simulink model "Transition"  (R2019a)
settings: Solver=VariableStepAuto  StartTime=0.0  StopTime=40  RelTol=1e-3
values from neighbouring files (symbols this model uses):
  agent = rlDDPGAgent(actor,critic,agentOptions)    [Agent.m]    (also in Bigger_Agent.m = agent.saved_agent; Multirotor_Agent.m = rlDDPGAgent(actor,critic,agentOpts); Transition_Agent.m = rlDDPGAgent(actor,critic,agentOpts))
  Ts = 0.4    [Agent.m]    (also in Bigger_Agent.m = 0.3; Multirotor_Agent.m = 0.3; Transition_Agent.m = 0.3)
libraries: simulink x14, simulink_extras x5, sharedutil x3, aerolibasang x2, shared6dof x1, aerolibadyn x1
(part 1 of 2)
settings Model: Creator=Michael  LastModifiedBy=admin
settings SolverCC: ZeroCrossAlgorithm=Adaptive
settings DebuggingCC: IgnoredZcDiagnostic=none

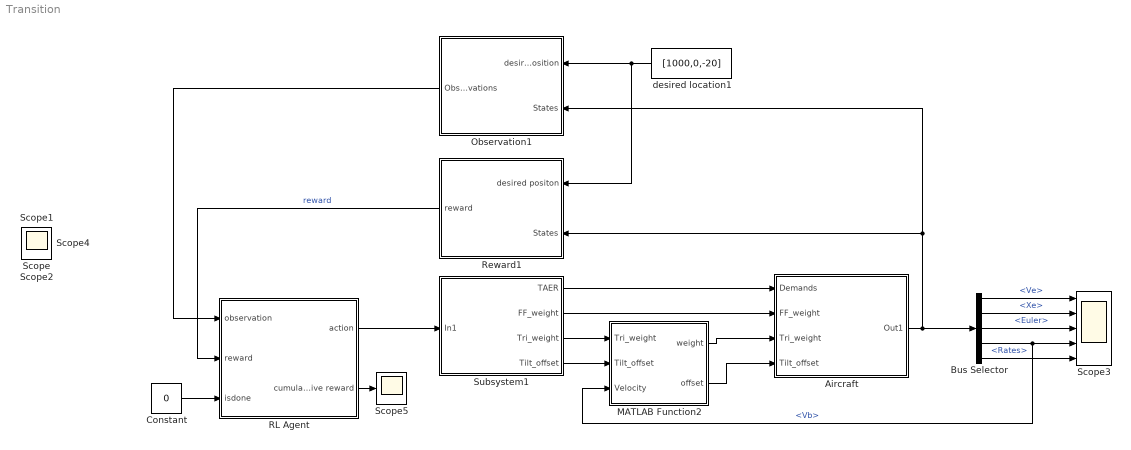
== system Transition ==
  "Aircraft " : Subsystem
  Bus Selector : BusSelector  OutputSignals=Ve,Xe,Euler,Vb,Rates
  Constant : Constant  Value=0
  MATLAB Function2 : MATLAB Function  TreatAsAtomicUnit=on
  Observation1 : Subsystem
  RL Agent : Subsystem  AncestorBlock=rllib/RL Agent  mask(RL Agent){Agent=agent, ProvideReward=on, ProvideIsDone=on, ProvideCumRwd=off, TreatAsDirectFeedthrough=on, CollectLoggedSignals=on, CollectModelStates=on}
      mask prompts: Agent "rl:block:RLAgentAgentPrompt"; ProvideReward "rl:block:RLAgentProvideRewardPrompt"; ProvideIsDone "rl:block:RLAgentProvideIsDonePrompt"; ProvideCumRwd "rl:block:RLAgentProvideCumRwdPrompt"; TreatAsDirectFeedthrough "rl:block:RLAgentDirectFeedthroughPrompt"; CollectLoggedSignals "rl:block:RLAgentCollectLoggedSignalsPrompt"; CollectModelStates "rl:block:RLAgentCollectModelStatesPrompt"
      mask help: rl:block:RLAgentDescription
      mask init:
      | agentmaskinit(gcb);
      mask Help: eval('rl.util.guihelp(''rlAgentBlock'')')
      mask DialogControl BDCollapsible Prompt: Block Diagram
      mask DialogControl AgentGroup Prompt: rl:block:RLAgentAgentGroupPrompt
      mask DialogControl Agent Prompt: Agent object
      mask DialogControl Agent Tooltip: rl:block:RLAgentAgentTooltip
      mask DialogControl PortGroup Prompt: rl:block:RLAgentPortsGroupPrompt
      mask DialogControl ProvideReward Prompt: Provide reward signal
      mask DialogControl ProvideReward Tooltip: rl:block:RLAgentProvideRewardTooltip
      mask DialogControl ProvideIsDone Prompt: Provide isdone signal
      mask DialogControl ProvideIsDone Tooltip: rl:block:RLAgentProvideIsDoneTooltip
      mask DialogControl ProvideCumRwd Prompt: Output cumulative reward signal
      mask DialogControl ProvideCumRwd Tooltip: rl:block:RLAgentProvideCumRwdTooltip
      mask DialogControl DirectFeedThroughGroup Prompt: rl:block:RLAgentDirectFeedthroughGroupPrompt
      mask DialogControl TreatAsDirectFeedthrough Prompt: Treat inputs as direct feedthrough
      mask DialogControl TreatAsDirectFeedthrough Tooltip: rl:block:RLAgentDirectFeedthroughTooltip
      mask DialogControl DataGroup Prompt: rl:block:RLAgentDataGroupPrompt
      mask DialogControl CollectLoggedSignals Prompt: Provide logged signals to agent
      mask DialogControl CollectLoggedSignals Tooltip: rl:block:RLAgentCollectLoggedSignalsTooltip
      mask DialogControl CollectModelStates Prompt: Provide model states to agent
      mask DialogControl CollectModelStates Tooltip: rl:block:RLAgentCollectModelStatesTooltip
  Reward1 : Subsystem
  Scope3 : Scope  NumInputPorts=5
  Scope{,1..2,4..5} (5 alike) : Scope
  Subsystem1 : Subsystem
  desired location1 : Constant  Value=[1000,0,-20]
  wires:
  Subsystem1/1(TAER) -> "Aircraft "/1(Demands)
  Bus Selector/1 -> Scope3/1  "<Ve>"
  Bus Selector/2 -> Scope3/2  "<Xe>"
  Bus Selector/3 -> Scope3/3  "<Euler>"
  Bus Selector/4 -> MATLAB Function2/3(Velocity), Scope3/4  "<Vb>"
  Bus Selector/5 -> Scope3/5  "<Rates>"
  RL Agent/1(action) -> Subsystem1/1(In1)
  Observation1/1("Observations ") -> RL Agent/1(observation)
  Reward1/1(reward) -> RL Agent/2(reward)  "reward"
  "Aircraft "/1(Out1) -> Bus Selector/1, Observation1/2(States), Reward1/2(States)
  Subsystem1/2(FF_weight) -> "Aircraft "/2(FF_weight)
  Subsystem1/3(Tri_weight) -> MATLAB Function2/1(Tri_weight)
  Subsystem1/4(Tilt_offset) -> MATLAB Function2/2(Tilt_offset)
  MATLAB Function2/1(weight) -> "Aircraft "/3(Tri_weight)
  MATLAB Function2/2(offset) -> "Aircraft "/4(Tilt_offset)
  Constant/1 -> RL Agent/3(isdone)
  RL Agent/2(cumulative reward) -> Scope5/1
  desired location1/1 -> Reward1/1(desired positon), Observation1/1(desired position)

== system Transition/Aircraft  ==
  Demands : Inport
  FF_weight : Inport  Port=2
  Tri_weight : Inport  Port=3
  Tilt_offset : Inport  Port=4
  FFController1 : Subsystem
  FF_Attitude Controller1 : Subsystem
  Flight Dynamics : Subsystem  mask{mass=7}
  Subsystem1 : Subsystem
  Tri_Attitude Controller : Subsystem
  Tri_Rates_Controller : Subsystem
  Out1 : Outport
  wires:
  Flight Dynamics/1(States) -> Tri_Attitude Controller/2("States "), FF_Attitude Controller1/2("States "), Tri_Rates_Controller/2("States "), FFController1/2("States "), Out1/1
  Tri_Rates_Controller/1(Control) -> Subsystem1/5(Tri Control)
  Tri_Attitude Controller/1(Rate Demand) -> Tri_Rates_Controller/1(Demand)
  Subsystem1/1(Out1) -> Flight Dynamics/1(Control)
  FFController1/1(Control) -> Subsystem1/1(FF Control)
  FF_weight/1 -> Subsystem1/2(FF Weight)
  Tri_weight/1 -> Subsystem1/3("Tri Weight ")
  FF_Attitude Controller1/1(Rate Demand) -> FFController1/1(Demand)
  Demands/1 -> Tri_Attitude Controller/1("Demand "), FF_Attitude Controller1/1("Demand ")
  Tilt_offset/1 -> Subsystem1/4(Tilt_offset)

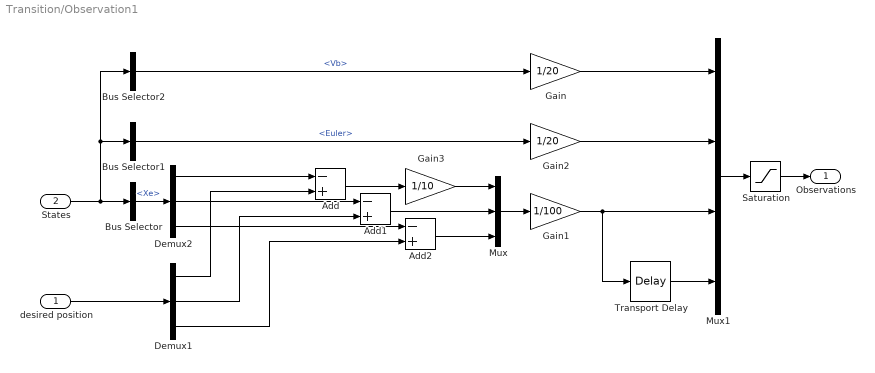
== system Transition/Observation1 ==
  desired position : Inport
  States : Inport  Port=2
  Add : Sum  Inputs=-+
  Add1 : Sum  Inputs=-+
  Add2 : Sum  Inputs=-+
  Bus Selector : BusSelector  OutputSignals=Xe
  Bus Selector1 : BusSelector  OutputSignals=Euler
  Bus Selector2 : BusSelector  OutputSignals=Vb
  Demux1 : Demux  Outputs=3
  Demux2 : Demux  Outputs=3
  Gain : Gain  Gain=1/20
  Gain1 : Gain  Gain=1/100
  Gain2 : Gain  Gain=1/20
  Gain3 : Gain  Gain=1/10
  Mux : Mux  Inputs=3
  Mux1 : Mux
  Saturation : Saturate  UpperLimit=1  LowerLimit=-1
  Transport Delay : TransportDelay  DelayTime=Ts
  "Observations " : Outport
  wires:
  desired position/1 -> Demux1/1
  Mux1/1 -> Saturation/1
  Add/1 -> Gain3/1
  Demux1/3 -> Add2/2
  Add2/1 -> Mux/3
  Add1/1 -> Mux/2
  Demux2/3 -> Add2/1
  Bus Selector/1 -> Demux2/1  "<Xe>"
  Demux1/2 -> Add1/2
  Demux2/1 -> Add/1
  Demux2/2 -> Add1/1
  Demux1/1 -> Add/2
  Bus Selector1/1 -> Gain2/1  "<Euler>"
  States/1 -> Bus Selector2/1, Bus Selector1/1, Bus Selector/1
  Bus Selector2/1 -> Gain/1  "<Vb>"
  Mux/1 -> Gain1/1
  Gain/1 -> Mux1/1
  Gain2/1 -> Mux1/2
  Gain1/1 -> Transport Delay/1, Mux1/3
  Transport Delay/1 -> Mux1/4
  Saturation/1 -> "Observations "/1
  Gain3/1 -> Mux/1

== system Transition/RL Agent ==
  observation : Inport
  reward : Inport  Port=2
  isdone : Inport  Port=3
  AgentWrapper : MATLABSystem  System=AgentWrapper  ModelName=Transition  AgentObjectName=Agent  BlockPath=Transition/RL Agent/AgentWrapper  TreatAsDirectFeedthrough=true  IsRewardProvided=true  IsIsDoneProvided=true  CollectLoggedSignals=true  CollectModelStates=true
      mask Type: AgentWrapper
      mask Display:
      | disp('AgentWrapper');
      | port_label('input',1,'observation');
      | port_label('input',2,'reward');
      | port_label('input',3,'isdone');
      | port_label('output',1,'action');
  accumulate_reward : Subsystem
  cumulative_reward : Terminator
  action : Outport
  cumulative reward : Outport  Port=2
  wires:
  AgentWrapper/1 -> action/1
  accumulate_reward/1(cumulative_reward) -> cumulative_reward/1, cumulative reward/1
  observation/1 -> AgentWrapper/1
  reward/1 -> accumulate_reward/1(reward), AgentWrapper/2
  isdone/1 -> AgentWrapper/3

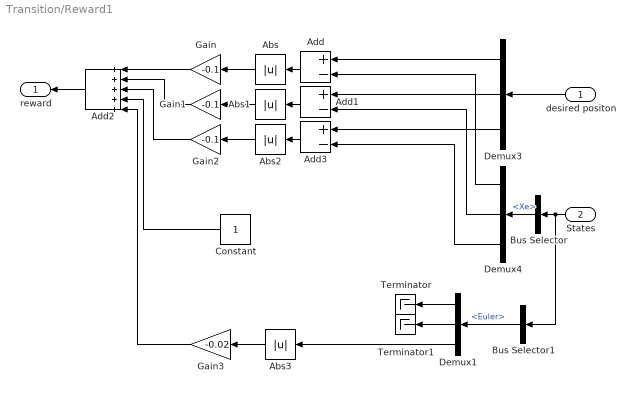
== system Transition/Reward1 ==
  desired positon : Inport
  States : Inport  Port=2
  Abs{,1..3} (4 alike) : Abs
  Add : Sum  Inputs=+-
  Add1 : Sum  Inputs=+-
  Add2 : Sum  Inputs=+++++
  Add3 : Sum  Inputs=+-
  Bus Selector : BusSelector  OutputSignals=Xe
  Bus Selector1 : BusSelector  OutputSignals=Euler
  Constant : Constant
  Demux1 : Demux  Outputs=3
  Demux3 : Demux  Outputs=3
  Demux4 : Demux  Outputs=3
  Gain : Gain  Gain=-0.1
  Gain1 : Gain  Gain=-0.1
  Gain2 : Gain  Gain=-0.1
  Gain3 : Gain  Gain=-0.02
  Terminator : Terminator
  Terminator1 : Terminator
  reward : Outport
  wires:
  Demux3/1 -> Add/1
  desired positon/1 -> Demux3/1
  Bus Selector/1 -> Demux4/1  "<Xe>"
  Add/1 -> Abs/1
  Demux4/1 -> Add/2
  Abs/1 -> Gain/1
  Demux3/2 -> Add1/1
  Demux4/2 -> Add1/2
  Abs1/1 -> Gain1/1
  Add1/1 -> Abs1/1
  Gain1/1 -> Add2/2
  Gain/1 -> Add2/1
  Add2/1 -> reward/1
  Gain2/1 -> Add2/3
  Add3/1 -> Abs2/1
  Abs2/1 -> Gain2/1
  Demux3/3 -> Add3/1
  Demux4/3 -> Add3/2
  Constant/1 -> Add2/4
  Bus Selector1/1 -> Demux1/1  "<Euler>"
  States/1 -> Bus Selector1/1, Bus Selector/1
  Demux1/1 -> Terminator/1
  Demux1/2 -> Terminator1/1
  Demux1/3 -> Abs3/1
  Abs3/1 -> Gain3/1
  Gain3/1 -> Add2/5

== system Transition/Subsystem1 ==
  In1 : Inport
  -1/1 to 0/1_1 : Subsystem
  -1/1 to 0/1_2 : Subsystem
  -1/1 to 0/1_3 : Subsystem
  Bus Creator : BusCreator  Inputs=4
  Constant : Constant  Value=0
  Demux1 : Demux  Outputs=6
  Gain4 : Gain  Gain=90
  TAER : Outport
  FF_weight : Outport  Port=2
  Tri_weight : Outport  Port=3
  Tilt_offset : Outport  Port=4
  wires:
  Demux1/2 -> Bus Creator/3  "Rd"
  Demux1/1 -> Bus Creator/2  "Xv"
  Demux1/3 -> Bus Creator/4  "Pd"
  -1/1 to 0/1_1/1(o) -> Gain4/1
  -1/1 to 0/1_3/1(o) -> FF_weight/1
  Gain4/1 -> Tilt_offset/1
  In1/1 -> Demux1/1
  Demux1/4 -> -1/1 to 0/1_1/1(<i>)
  Demux1/5 -> -1/1 to 0/1_2/1(<i>)
  Demux1/6 -> -1/1 to 0/1_3/1(<i>)
  -1/1 to 0/1_2/1(o) -> Tri_weight/1
  Constant/1 -> Bus Creator/1  "Yd"
  Bus Creator/1 -> TAER/1

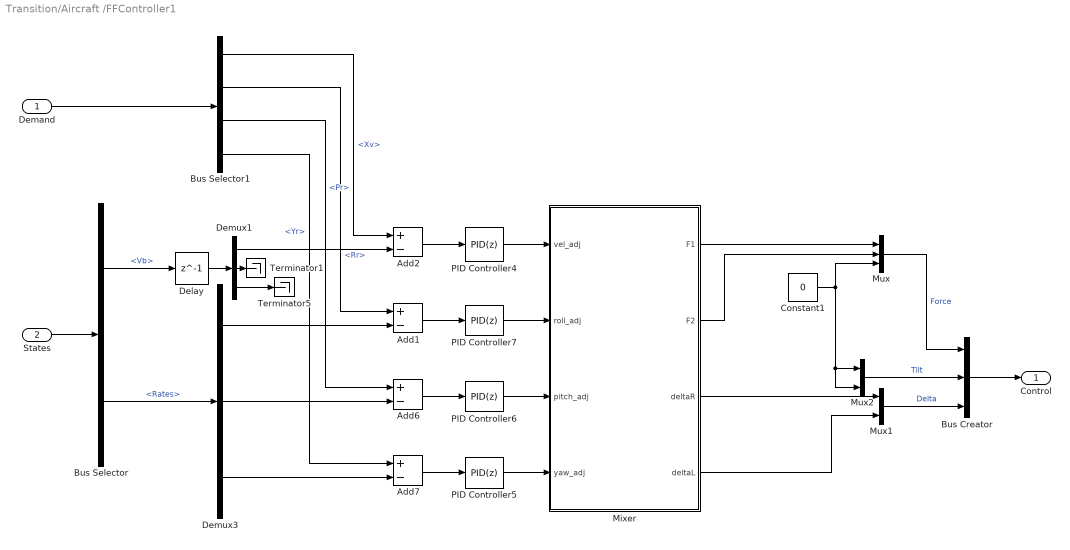
== system Transition/Aircraft /FFController1 ==
  Demand : Inport
  "States " : Inport  Port=2
  Add{1..2,6..7} (4 alike) : Sum  Inputs=+-
  Bus Creator : BusCreator  Inputs=3
  Bus Selector : BusSelector  OutputSignals=Vb,Rates
  Bus Selector1 : BusSelector  OutputSignals=Xv,Rr,Pr,Yr
  Constant1 : Constant  Value=0
  Delay : Delay  DelayLength=1  InitialCondition=0
  Demux1 : Demux  Outputs=3
  Demux3 : Demux  Outputs=3
  Mixer : Subsystem
  Mux : Mux  Inputs=3
  Mux1 : Mux  Inputs=2
  Mux2 : Mux  Inputs=2
  PID Controller4 : simulink/Continuous/PID Controller  Controller=PID  Form=Parallel  TimeDomain=Discrete-time  SampleTime=0.001  IntegratorMethod=Forward Euler  FilterMethod=Forward Euler  ControllerParametersSource=internal  P=30  I=0  D=1  UseFilter=on  N=21.8158810168648  TunerSelectOption=Transfer Function Based (PID Tuner App)  InitialConditionSource=internal  InitialConditionForIntegrator=0  InitialConditionForFilter=0  DifferentiatorICPrevScaledInput=0  ExternalReset=none  TrackingMode=off  Kt=1  LimitOutput=off  UpperSaturationLimit=inf  LowerSaturationLimit=-inf  LinearizeAsGain=on  AntiWindupMode=none  Kb=1  POutMin=[]  POutMax=[]  IOutMin=[]  IOutMax=[]  DOutMin=[]  DOutMax=[]  NOutMin=[]  NOutMax=[]  SumOutMin=[]  SumOutMax=[]  SaturationOutMin=[]  SaturationOutMax=[]  PParamMin=[]  PParamMax=[]  IParamMin=[]  IParamMax=[]  DParamMin=[]  DParamMax=[]  NParamMin=[]  NParamMax=[]  KbParamMin=[]  KbParamMax=[]  KtParamMin=[]  KtParamMax=[]  KbOutMin=[]  KbOutMax=[]  KtOutMin=[]  KtOutMax=[]  IntegratorOutMin=[]  IntegratorOutMax=[]  FilterOutMin=[]  FilterOutMax=[]  SumI1OutMin=[]  SumI1OutMax=[]  SumI2OutMin=[]  SumI2OutMax=[]  SumI3OutMin=[]  SumI3OutMax=[]  SumI4OutMin=[]  SumI4OutMax=[]  SumDOutMin=[]  SumDOutMax=[]  DifferentiatorOutMin=[]  DifferentiatorOutMax=[]  FilterDiffOutCoefMin=[]  FilterDiffOutCoefMax=[]  ReciprocalOutMin=[]  ReciprocalOutMax=[]  SumDenOutMin=[]  SumDenOutMax=[]  SumNumOutMin=[]  SumNumOutMax=[]  DivideOutMin=[]  DivideOutMax=[]  IntegratorContinuousStateAttributes=''  IntegratorStateMustResolveToSignalObject=off  IntegratorRTWStateStorageClass=Auto  FilterContinuousStateAttributes=''  FilterStateMustResolveToSignalObject=off  FilterRTWStateStorageClass=Auto  ParallelPVariant=InternalParameters  IdealPVariant=Disabled  IVariant=InternalParameters  DVariant=InternalParameters  IntegratorVariant=Discrete  SatVariant=Disabled  AWVariant=Passthrough  PCopyVariant=Disabled  TRVariant=Disabled  FdbkBlocksVariant=Forward  IdealPFdbkVariant=Disabled  SatFdbkVariant=Disabled  DerivativeFilterVariant=ForwardEulerFilter  NVariant=InternalParameters  NCopyVariant=Disabled  FilterICVariant=InternalICsFilter  IntegratorICVariant=InternalICs  ExternalResetVariant=Disabled  TRSumVariant=Passthrough  SumFdbkVariant=Disabled  SumVariant=Sum_PID
  PID Controller5 : simulink/Continuous/PID Controller  Controller=PID  Form=Parallel  TimeDomain=Discrete-time  SampleTime=0.001  IntegratorMethod=Forward Euler  FilterMethod=Forward Euler  ControllerParametersSource=internal  P=30  I=0.01  D=2  UseFilter=on  N=200  TunerSelectOption=Transfer Function Based (PID Tuner App)  InitialConditionSource=internal  InitialConditionForIntegrator=0  InitialConditionForFilter=0  DifferentiatorICPrevScaledInput=0  ExternalReset=none  TrackingMode=off  Kt=1  LimitOutput=off  UpperSaturationLimit=inf  LowerSaturationLimit=-inf  LinearizeAsGain=on  AntiWindupMode=none  Kb=1  POutMin=[]  POutMax=[]  IOutMin=[]  IOutMax=[]  DOutMin=[]  DOutMax=[]  NOutMin=[]  NOutMax=[]  SumOutMin=[]  SumOutMax=[]  SaturationOutMin=[]  SaturationOutMax=[]  PParamMin=[]  PParamMax=[]  IParamMin=[]  IParamMax=[]  DParamMin=[]  DParamMax=[]  NParamMin=[]  NParamMax=[]  KbParamMin=[]  KbParamMax=[]  KtParamMin=[]  KtParamMax=[]  KbOutMin=[]  KbOutMax=[]  KtOutMin=[]  KtOutMax=[]  IntegratorOutMin=[]  IntegratorOutMax=[]  FilterOutMin=[]  FilterOutMax=[]  SumI1OutMin=[]  SumI1OutMax=[]  SumI2OutMin=[]  SumI2OutMax=[]  SumI3OutMin=[]  SumI3OutMax=[]  SumI4OutMin=[]  SumI4OutMax=[]  SumDOutMin=[]  SumDOutMax=[]  DifferentiatorOutMin=[]  DifferentiatorOutMax=[]  FilterDiffOutCoefMin=[]  FilterDiffOutCoefMax=[]  ReciprocalOutMin=[]  ReciprocalOutMax=[]  SumDenOutMin=[]  SumDenOutMax=[]  SumNumOutMin=[]  SumNumOutMax=[]  DivideOutMin=[]  DivideOutMax=[]  IntegratorContinuousStateAttributes=''  IntegratorStateMustResolveToSignalObject=off  IntegratorRTWStateStorageClass=Auto  FilterContinuousStateAttributes=''  FilterStateMustResolveToSignalObject=off  FilterRTWStateStorageClass=Auto  ParallelPVariant=InternalParameters  IdealPVariant=Disabled  IVariant=InternalParameters  DVariant=InternalParameters  IntegratorVariant=Discrete  SatVariant=Disabled  AWVariant=Passthrough  PCopyVariant=Disabled  TRVariant=Disabled  FdbkBlocksVariant=Forward  IdealPFdbkVariant=Disabled  SatFdbkVariant=Disabled  DerivativeFilterVariant=ForwardEulerFilter  NVariant=InternalParameters  NCopyVariant=Disabled  FilterICVariant=InternalICsFilter  IntegratorICVariant=InternalICs  ExternalResetVariant=Disabled  TRSumVariant=Passthrough  SumFdbkVariant=Disabled  SumVariant=Sum_PID
  PID Controller6 : simulink/Continuous/PID Controller  Controller=PID  Form=Parallel  TimeDomain=Discrete-time  SampleTime=0.001  IntegratorMethod=Forward Euler  FilterMethod=Forward Euler  ControllerParametersSource=internal  P=40  I=0.01  D=2  UseFilter=on  N=200  TunerSelectOption=Transfer Function Based (PID Tuner App)  InitialConditionSource=internal  InitialConditionForIntegrator=0  InitialConditionForFilter=0  DifferentiatorICPrevScaledInput=0  ExternalReset=none  TrackingMode=off  Kt=1  LimitOutput=off  UpperSaturationLimit=inf  LowerSaturationLimit=-inf  LinearizeAsGain=on  AntiWindupMode=none  Kb=1  POutMin=[]  POutMax=[]  IOutMin=[]  IOutMax=[]  DOutMin=[]  DOutMax=[]  NOutMin=[]  NOutMax=[]  SumOutMin=[]  SumOutMax=[]  SaturationOutMin=[]  SaturationOutMax=[]  PParamMin=[]  PParamMax=[]  IParamMin=[]  IParamMax=[]  DParamMin=[]  DParamMax=[]  NParamMin=[]  NParamMax=[]  KbParamMin=[]  KbParamMax=[]  KtParamMin=[]  KtParamMax=[]  KbOutMin=[]  KbOutMax=[]  KtOutMin=[]  KtOutMax=[]  IntegratorOutMin=[]  IntegratorOutMax=[]  FilterOutMin=[]  FilterOutMax=[]  SumI1OutMin=[]  SumI1OutMax=[]  SumI2OutMin=[]  SumI2OutMax=[]  SumI3OutMin=[]  SumI3OutMax=[]  SumI4OutMin=[]  SumI4OutMax=[]  SumDOutMin=[]  SumDOutMax=[]  DifferentiatorOutMin=[]  DifferentiatorOutMax=[]  FilterDiffOutCoefMin=[]  FilterDiffOutCoefMax=[]  ReciprocalOutMin=[]  ReciprocalOutMax=[]  SumDenOutMin=[]  SumDenOutMax=[]  SumNumOutMin=[]  SumNumOutMax=[]  DivideOutMin=[]  DivideOutMax=[]  IntegratorContinuousStateAttributes=''  IntegratorStateMustResolveToSignalObject=off  IntegratorRTWStateStorageClass=Auto  FilterContinuousStateAttributes=''  FilterStateMustResolveToSignalObject=off  FilterRTWStateStorageClass=Auto  ParallelPVariant=InternalParameters  IdealPVariant=Disabled  IVariant=InternalParameters  DVariant=InternalParameters  IntegratorVariant=Discrete  SatVariant=Disabled  AWVariant=Passthrough  PCopyVariant=Disabled  TRVariant=Disabled  FdbkBlocksVariant=Forward  IdealPFdbkVariant=Disabled  SatFdbkVariant=Disabled  DerivativeFilterVariant=ForwardEulerFilter  NVariant=InternalParameters  NCopyVariant=Disabled  FilterICVariant=InternalICsFilter  IntegratorICVariant=InternalICs  ExternalResetVariant=Disabled  TRSumVariant=Passthrough  SumFdbkVariant=Disabled  SumVariant=Sum_PID
  PID Controller7 : simulink/Continuous/PID Controller  Controller=PID  Form=Parallel  TimeDomain=Discrete-time  SampleTime=0.001  IntegratorMethod=Forward Euler  FilterMethod=Forward Euler  ControllerParametersSource=internal  P=20  I=0.01  D=2  UseFilter=on  N=200  TunerSelectOption=Transfer Function Based (PID Tuner App)  InitialConditionSource=internal  InitialConditionForIntegrator=0  InitialConditionForFilter=0  DifferentiatorICPrevScaledInput=0  ExternalReset=none  TrackingMode=off  Kt=1  LimitOutput=off  UpperSaturationLimit=inf  LowerSaturationLimit=-inf  LinearizeAsGain=on  AntiWindupMode=none  Kb=1  POutMin=[]  POutMax=[]  IOutMin=[]  IOutMax=[]  DOutMin=[]  DOutMax=[]  NOutMin=[]  NOutMax=[]  SumOutMin=[]  SumOutMax=[]  SaturationOutMin=[]  SaturationOutMax=[]  PParamMin=[]  PParamMax=[]  IParamMin=[]  IParamMax=[]  DParamMin=[]  DParamMax=[]  NParamMin=[]  NParamMax=[]  KbParamMin=[]  KbParamMax=[]  KtParamMin=[]  KtParamMax=[]  KbOutMin=[]  KbOutMax=[]  KtOutMin=[]  KtOutMax=[]  IntegratorOutMin=[]  IntegratorOutMax=[]  FilterOutMin=[]  FilterOutMax=[]  SumI1OutMin=[]  SumI1OutMax=[]  SumI2OutMin=[]  SumI2OutMax=[]  SumI3OutMin=[]  SumI3OutMax=[]  SumI4OutMin=[]  SumI4OutMax=[]  SumDOutMin=[]  SumDOutMax=[]  DifferentiatorOutMin=[]  DifferentiatorOutMax=[]  FilterDiffOutCoefMin=[]  FilterDiffOutCoefMax=[]  ReciprocalOutMin=[]  ReciprocalOutMax=[]  SumDenOutMin=[]  SumDenOutMax=[]  SumNumOutMin=[]  SumNumOutMax=[]  DivideOutMin=[]  DivideOutMax=[]  IntegratorContinuousStateAttributes=''  IntegratorStateMustResolveToSignalObject=off  IntegratorRTWStateStorageClass=Auto  FilterContinuousStateAttributes=''  FilterStateMustResolveToSignalObject=off  FilterRTWStateStorageClass=Auto  ParallelPVariant=InternalParameters  IdealPVariant=Disabled  IVariant=InternalParameters  DVariant=InternalParameters  IntegratorVariant=Discrete  SatVariant=Disabled  AWVariant=Passthrough  PCopyVariant=Disabled  TRVariant=Disabled  FdbkBlocksVariant=Forward  IdealPFdbkVariant=Disabled  SatFdbkVariant=Disabled  DerivativeFilterVariant=ForwardEulerFilter  NVariant=InternalParameters  NCopyVariant=Disabled  FilterICVariant=InternalICsFilter  IntegratorICVariant=InternalICs  ExternalResetVariant=Disabled  TRSumVariant=Passthrough  SumFdbkVariant=Disabled  SumVariant=Sum_PID
  Terminator1 : Terminator
  Terminator5 : Terminator
  Control : Outport
  wires:
  Mixer/1(F1) -> Mux/1
  Mixer/2(F2) -> Mux/2
  Mixer/3(deltaR) -> Mux1/1
  Mixer/4(deltaL) -> Mux1/2
  Mux1/1 -> Bus Creator/3  "Delta"
  Mux/1 -> Bus Creator/1  "Force"
  Constant1/1 -> Mux2/2, Mux2/1, Mux/3
  Mux2/1 -> Bus Creator/2  "Tilt"
  Bus Creator/1 -> Control/1
  PID Controller7/1 -> Mixer/2(roll_adj)
  Add1/1 -> PID Controller7/1
  Bus Selector1/3 -> Add6/1  "<Pr>"
  Add6/1 -> PID Controller6/1
  PID Controller6/1 -> Mixer/3(pitch_adj)
  Add7/1 -> PID Controller5/1
  Bus Selector1/4 -> Add7/1  "<Yr>"
  Demux3/2 -> Add6/2
  Demux1/1 -> Add2/2
  Demux1/2 -> Terminator1/1
  Bus Selector/2 -> Demux3/1  "<Rates>"
  Bus Selector1/2 -> Add1/1  "<Rr>"
  Bus Selector/1 -> Delay/1  "<Vb>"
  Add2/1 -> PID Controller4/1
  Demux3/3 -> Add7/2
  PID Controller5/1 -> Mixer/4(yaw_adj)
  PID Controller4/1 -> Mixer/1(vel_adj)
  Demux3/1 -> Add1/2
  Demand/1 -> Bus Selector1/1
  Bus Selector1/1 -> Add2/1  "<Xv>"
  "States "/1 -> Bus Selector/1
  Demux1/3 -> Terminator5/1
  Delay/1 -> Demux1/1

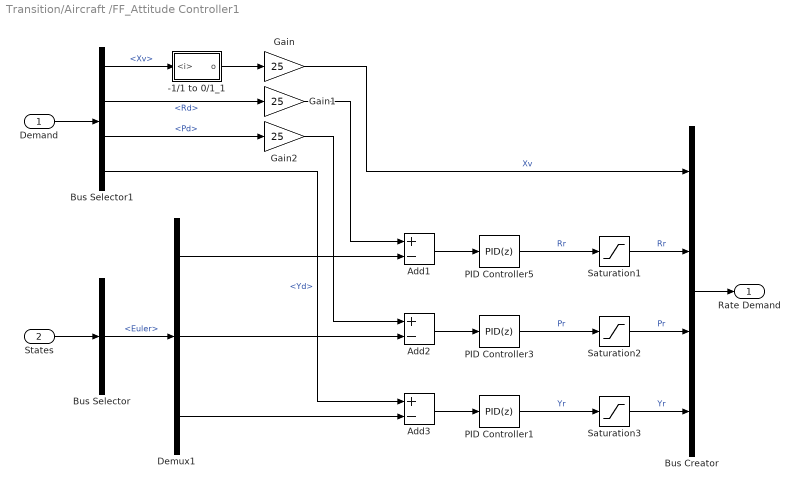
== system Transition/Aircraft /FF_Attitude Controller1 ==
  "Demand " : Inport
  "States " : Inport  Port=2
  -1/1 to 0/1_1 : Subsystem
  Add1 : Sum  Inputs=+-
  Add2 : Sum  Inputs=+-
  Add3 : Sum  Inputs=+-
  Bus Creator : BusCreator  Inputs=4
  Bus Selector : BusSelector  OutputSignals=Euler
  Bus Selector1 : BusSelector  OutputSignals=Xv,Rd,Pd,Yd
  Demux1 : Demux  Outputs=3
  Gain : Gain  Gain=25
  Gain1 : Gain  Gain=25
  Gain2 : Gain  Gain=25
  PID Controller1 : simulink/Continuous/PID Controller  Controller=PID  Form=Parallel  TimeDomain=Discrete-time  SampleTime=0.001  IntegratorMethod=Forward Euler  FilterMethod=Forward Euler  ControllerParametersSource=internal  P=3  I=0  D=0  UseFilter=on  N=200  TunerSelectOption=Transfer Function Based (PID Tuner App)  InitialConditionSource=internal  InitialConditionForIntegrator=0  InitialConditionForFilter=0  DifferentiatorICPrevScaledInput=0  ExternalReset=none  TrackingMode=off  Kt=1  LimitOutput=off  UpperSaturationLimit=inf  LowerSaturationLimit=-inf  LinearizeAsGain=on  AntiWindupMode=none  Kb=1  POutMin=[]  POutMax=[]  IOutMin=[]  IOutMax=[]  DOutMin=[]  DOutMax=[]  NOutMin=[]  NOutMax=[]  SumOutMin=[]  SumOutMax=[]  SaturationOutMin=[]  SaturationOutMax=[]  PParamMin=[]  PParamMax=[]  IParamMin=[]  IParamMax=[]  DParamMin=[]  DParamMax=[]  NParamMin=[]  NParamMax=[]  KbParamMin=[]  KbParamMax=[]  KtParamMin=[]  KtParamMax=[]  KbOutMin=[]  KbOutMax=[]  KtOutMin=[]  KtOutMax=[]  IntegratorOutMin=[]  IntegratorOutMax=[]  FilterOutMin=[]  FilterOutMax=[]  SumI1OutMin=[]  SumI1OutMax=[]  SumI2OutMin=[]  SumI2OutMax=[]  SumI3OutMin=[]  SumI3OutMax=[]  SumI4OutMin=[]  SumI4OutMax=[]  SumDOutMin=[]  SumDOutMax=[]  DifferentiatorOutMin=[]  DifferentiatorOutMax=[]  FilterDiffOutCoefMin=[]  FilterDiffOutCoefMax=[]  ReciprocalOutMin=[]  ReciprocalOutMax=[]  SumDenOutMin=[]  SumDenOutMax=[]  SumNumOutMin=[]  SumNumOutMax=[]  DivideOutMin=[]  DivideOutMax=[]  IntegratorContinuousStateAttributes=''  IntegratorStateMustResolveToSignalObject=off  IntegratorRTWStateStorageClass=Auto  FilterContinuousStateAttributes=''  FilterStateMustResolveToSignalObject=off  FilterRTWStateStorageClass=Auto  ParallelPVariant=InternalParameters  IdealPVariant=Disabled  IVariant=InternalParameters  DVariant=InternalParameters  IntegratorVariant=Discrete  SatVariant=Disabled  AWVariant=Passthrough  PCopyVariant=Disabled  TRVariant=Disabled  FdbkBlocksVariant=Forward  IdealPFdbkVariant=Disabled  SatFdbkVariant=Disabled  DerivativeFilterVariant=ForwardEulerFilter  NVariant=InternalParameters  NCopyVariant=Disabled  FilterICVariant=InternalICsFilter  IntegratorICVariant=InternalICs  ExternalResetVariant=Disabled  TRSumVariant=Passthrough  SumFdbkVariant=Disabled  SumVariant=Sum_PID
  PID Controller3 : simulink/Continuous/PID Controller  Controller=PID  Form=Parallel  TimeDomain=Discrete-time  SampleTime=0.001  IntegratorMethod=Forward Euler  FilterMethod=Forward Euler  ControllerParametersSource=internal  P=40  I=0.1  D=0.5  UseFilter=on  N=200  TunerSelectOption=Transfer Function Based (PID Tuner App)  InitialConditionSource=internal  InitialConditionForIntegrator=0  InitialConditionForFilter=0  DifferentiatorICPrevScaledInput=0  ExternalReset=none  TrackingMode=off  Kt=1  LimitOutput=off  UpperSaturationLimit=inf  LowerSaturationLimit=-inf  LinearizeAsGain=on  AntiWindupMode=none  Kb=1  POutMin=[]  POutMax=[]  IOutMin=[]  IOutMax=[]  DOutMin=[]  DOutMax=[]  NOutMin=[]  NOutMax=[]  SumOutMin=[]  SumOutMax=[]  SaturationOutMin=[]  SaturationOutMax=[]  PParamMin=[]  PParamMax=[]  IParamMin=[]  IParamMax=[]  DParamMin=[]  DParamMax=[]  NParamMin=[]  NParamMax=[]  KbParamMin=[]  KbParamMax=[]  KtParamMin=[]  KtParamMax=[]  KbOutMin=[]  KbOutMax=[]  KtOutMin=[]  KtOutMax=[]  IntegratorOutMin=[]  IntegratorOutMax=[]  FilterOutMin=[]  FilterOutMax=[]  SumI1OutMin=[]  SumI1OutMax=[]  SumI2OutMin=[]  SumI2OutMax=[]  SumI3OutMin=[]  SumI3OutMax=[]  SumI4OutMin=[]  SumI4OutMax=[]  SumDOutMin=[]  SumDOutMax=[]  DifferentiatorOutMin=[]  DifferentiatorOutMax=[]  FilterDiffOutCoefMin=[]  FilterDiffOutCoefMax=[]  ReciprocalOutMin=[]  ReciprocalOutMax=[]  SumDenOutMin=[]  SumDenOutMax=[]  SumNumOutMin=[]  SumNumOutMax=[]  DivideOutMin=[]  DivideOutMax=[]  IntegratorContinuousStateAttributes=''  IntegratorStateMustResolveToSignalObject=off  IntegratorRTWStateStorageClass=Auto  FilterContinuousStateAttributes=''  FilterStateMustResolveToSignalObject=off  FilterRTWStateStorageClass=Auto  ParallelPVariant=InternalParameters  IdealPVariant=Disabled  IVariant=InternalParameters  DVariant=InternalParameters  IntegratorVariant=Discrete  SatVariant=Disabled  AWVariant=Passthrough  PCopyVariant=Disabled  TRVariant=Disabled  FdbkBlocksVariant=Forward  IdealPFdbkVariant=Disabled  SatFdbkVariant=Disabled  DerivativeFilterVariant=ForwardEulerFilter  NVariant=InternalParameters  NCopyVariant=Disabled  FilterICVariant=InternalICsFilter  IntegratorICVariant=InternalICs  ExternalResetVariant=Disabled  TRSumVariant=Passthrough  SumFdbkVariant=Disabled  SumVariant=Sum_PID
  PID Controller5 : simulink/Continuous/PID Controller  Controller=PID  Form=Parallel  TimeDomain=Discrete-time  SampleTime=0.001  IntegratorMethod=Forward Euler  FilterMethod=Forward Euler  ControllerParametersSource=internal  P=20  I=0.1  D=0.5  UseFilter=on  N=200  TunerSelectOption=Transfer Function Based (PID Tuner App)  InitialConditionSource=internal  InitialConditionForIntegrator=0  InitialConditionForFilter=0  DifferentiatorICPrevScaledInput=0  ExternalReset=none  TrackingMode=off  Kt=1  LimitOutput=off  UpperSaturationLimit=inf  LowerSaturationLimit=-inf  LinearizeAsGain=on  AntiWindupMode=none  Kb=1  POutMin=[]  POutMax=[]  IOutMin=[]  IOutMax=[]  DOutMin=[]  DOutMax=[]  NOutMin=[]  NOutMax=[]  SumOutMin=[]  SumOutMax=[]  SaturationOutMin=[]  SaturationOutMax=[]  PParamMin=[]  PParamMax=[]  IParamMin=[]  IParamMax=[]  DParamMin=[]  DParamMax=[]  NParamMin=[]  NParamMax=[]  KbParamMin=[]  KbParamMax=[]  KtParamMin=[]  KtParamMax=[]  KbOutMin=[]  KbOutMax=[]  KtOutMin=[]  KtOutMax=[]  IntegratorOutMin=[]  IntegratorOutMax=[]  FilterOutMin=[]  FilterOutMax=[]  SumI1OutMin=[]  SumI1OutMax=[]  SumI2OutMin=[]  SumI2OutMax=[]  SumI3OutMin=[]  SumI3OutMax=[]  SumI4OutMin=[]  SumI4OutMax=[]  SumDOutMin=[]  SumDOutMax=[]  DifferentiatorOutMin=[]  DifferentiatorOutMax=[]  FilterDiffOutCoefMin=[]  FilterDiffOutCoefMax=[]  ReciprocalOutMin=[]  ReciprocalOutMax=[]  SumDenOutMin=[]  SumDenOutMax=[]  SumNumOutMin=[]  SumNumOutMax=[]  DivideOutMin=[]  DivideOutMax=[]  IntegratorContinuousStateAttributes=''  IntegratorStateMustResolveToSignalObject=off  IntegratorRTWStateStorageClass=Auto  FilterContinuousStateAttributes=''  FilterStateMustResolveToSignalObject=off  FilterRTWStateStorageClass=Auto  ParallelPVariant=InternalParameters  IdealPVariant=Disabled  IVariant=InternalParameters  DVariant=InternalParameters  IntegratorVariant=Discrete  SatVariant=Disabled  AWVariant=Passthrough  PCopyVariant=Disabled  TRVariant=Disabled  FdbkBlocksVariant=Forward  IdealPFdbkVariant=Disabled  SatFdbkVariant=Disabled  DerivativeFilterVariant=ForwardEulerFilter  NVariant=InternalParameters  NCopyVariant=Disabled  FilterICVariant=InternalICsFilter  IntegratorICVariant=InternalICs  ExternalResetVariant=Disabled  TRSumVariant=Passthrough  SumFdbkVariant=Disabled  SumVariant=Sum_PID
  Saturation1 : Saturate  UpperLimit=25  LowerLimit=-25  LinearizeAsGain=off
  Saturation2 : Saturate  UpperLimit=15  LowerLimit=-15  LinearizeAsGain=off
  Saturation3 : Saturate  UpperLimit=30  LowerLimit=-30  LinearizeAsGain=off
  Rate Demand : Outport
  wires:
  Add2/1 -> PID Controller3/1
  Add3/1 -> PID Controller1/1
  Add1/1 -> PID Controller5/1
  PID Controller5/1 -> Saturation1/1  "Rr"
  PID Controller1/1 -> Saturation3/1  "Yr"
  PID Controller3/1 -> Saturation2/1  "Pr"
  Bus Selector1/3 -> Gain2/1  "<Pd>"
  Bus Selector1/2 -> Gain1/1  "<Rd>"
  Demux1/1 -> Add1/2
  Demux1/2 -> Add2/2
  "States "/1 -> Bus Selector/1
  Bus Selector/1 -> Demux1/1  "<Euler>"
  Demux1/3 -> Add3/2
  "Demand "/1 -> Bus Selector1/1
  Bus Creator/1 -> Rate Demand/1
  Gain/1 -> Bus Creator/1  "Xv"
  Saturation3/1 -> Bus Creator/4  "Yr"
  Saturation2/1 -> Bus Creator/3  "Pr"
  Saturation1/1 -> Bus Creator/2  "Rr"
  Bus Selector1/4 -> Add3/1  "<Yd>"
  Gain1/1 -> Add1/1
  Gain2/1 -> Add2/1
  Bus Selector1/1 -> -1/1 to 0/1_1/1(<i>)  "<Xv>"
  -1/1 to 0/1_1/1(o) -> Gain/1

== system Transition/Aircraft /Flight Dynamics ==
  Control : Inport
  6DOF (Euler Angles) : shared6dof/6DOF (Euler Angles)  units=Metric (MKS)  mtype=Fixed  rep=Euler Angles  xme_0=[0,0,0]  Vm_0=[0,0,0]  eul_0=[0,0,0]  pm_0=[0,0,0]  mass_0=mass  mass_e=0.5  mass_f=2.0  inertia=[1 0 0; 0 1 0;0 0 1]  inertia_e=eye(3)  inertia_f=2*eye(3)  k_quat=1.0  vre_flag=on  abi_flag=on  aMode=aMode  xme_statename=''  Vm_statename=''  eul_statename=''  quat_statename=''  pm_statename=''  mass_statename=''
      settings: SourceProductBaseCode=AE
  Add : Sum  Inputs=+++
  Add1 : Sum
  Aerodynamic Forces : Subsystem
  Bus Creator : BusCreator  Inputs=9
  Bus Selector1 : BusSelector  OutputSignals=Force,Tilt,Delta
  Gravitational Forces : Subsystem  mask{mass=mass}
  Propulsive Forces : Subsystem  mask{F=22}
      mask prompts: F "Max motor force"
  Radians to Degrees1 : simulink_extras/Transformations/Radians to Degrees
  Radians to Degrees2 : simulink_extras/Transformations/Radians to Degrees
  Scope : Scope
  Scope1 : Scope  NumInputPorts=3
  States : Outport
  wires:
  Aerodynamic Forces/2(M) -> Add1/2
  Bus Creator/1 -> States/1, Gravitational Forces/1(states), Aerodynamic Forces/2(Vb)
  6DOF (Euler Angles)/1 -> Bus Creator/1  "Ve"
  Gravitational Forces/1(Fg) -> Scope1/1, Add/1
  Aerodynamic Forces/1(F) -> Scope1/3, Add/3
  Propulsive Forces/1(F) -> Scope1/2, Add/2
  Add/1 -> 6DOF (Euler Angles)/1
  6DOF (Euler Angles)/2 -> Bus Creator/2  "Xe"
  Radians to Degrees1/1 -> Bus Creator/3  "Euler"
  6DOF (Euler Angles)/7 -> Bus Creator/7  "dWb/dt"
  6DOF (Euler Angles)/4 -> Bus Creator/4  "DCM"
  6DOF (Euler Angles)/5 -> Bus Creator/5  "Vb"
  6DOF (Euler Angles)/9 -> Bus Creator/9  "Abe"
  6DOF (Euler Angles)/8 -> Bus Creator/8  "Abb"
  Radians to Degrees2/1 -> Bus Creator/6  "Rates"
  Propulsive Forces/2(M) -> Add1/1
  Add1/1 -> 6DOF (Euler Angles)/2
  Control/1 -> Bus Selector1/1
  Bus Selector1/1 -> Scope/1, Propulsive Forces/1("F_M ")  "<Force>"
  Bus Selector1/3 -> Aerodynamic Forces/1(delta)  "<Delta>"
  Bus Selector1/2 -> Propulsive Forces/2(Tilt)  "<Tilt>"
  6DOF (Euler Angles)/3 -> Radians to Degrees1/1  "Euler"
  6DOF (Euler Angles)/6 -> Radians to Degrees2/1  "Rates"

== system Transition/Aircraft /Subsystem1 ==
  FF Control : Inport
  FF Weight : Inport  Port=2
  "Tri Weight " : Inport  Port=3
  Tilt_offset : Inport  Port=4
  Tri Control : Inport  Port=5
  Add : Subsystem
  Multiply_1 : Subsystem
  Multiply_2 : Subsystem
  Out1 : Outport
  wires:
  FF Weight/1 -> Multiply_1/1(Weight)
  Add/1(Out1) -> Out1/1
  "Tri Weight "/1 -> Multiply_2/1(Weight)
  Multiply_1/1(Control_out) -> Add/1(in_ff)
  Tri Control/1 -> Multiply_2/2(Control_in)
  FF Control/1 -> Multiply_1/2(Control_in)
  Tilt_offset/1 -> Add/3(Tilt_offset)
  Multiply_2/1(Control_out) -> Add/2(in_tri)

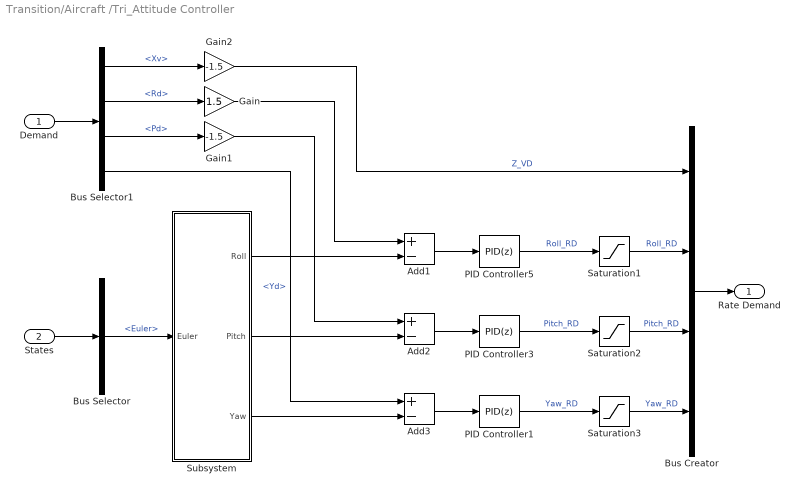
== system Transition/Aircraft /Tri_Attitude Controller ==
  "Demand " : Inport
  "States " : Inport  Port=2
  Add1 : Sum  Inputs=+-
  Add2 : Sum  Inputs=+-
  Add3 : Sum  Inputs=+-
  Bus Creator : BusCreator  Inputs=4
  Bus Selector : BusSelector  OutputSignals=Euler
  Bus Selector1 : BusSelector  OutputSignals=Xv,Rd,Pd,Yd
  Gain : Gain  Gain=1.5
  Gain1 : Gain  Gain=-1.5
  Gain2 : Gain  Gain=-1.5
  PID Controller1 : simulink/Continuous/PID Controller  Controller=PID  Form=Parallel  TimeDomain=Discrete-time  SampleTime=0.001  IntegratorMethod=Forward Euler  FilterMethod=Forward Euler  ControllerParametersSource=internal  P=3  I=0  D=0  UseFilter=on  N=200  TunerSelectOption=Transfer Function Based (PID Tuner App)  InitialConditionSource=internal  InitialConditionForIntegrator=0  InitialConditionForFilter=0  DifferentiatorICPrevScaledInput=0  ExternalReset=none  TrackingMode=off  Kt=1  LimitOutput=off  UpperSaturationLimit=inf  LowerSaturationLimit=-inf  LinearizeAsGain=on  AntiWindupMode=none  Kb=1  POutMin=[]  POutMax=[]  IOutMin=[]  IOutMax=[]  DOutMin=[]  DOutMax=[]  NOutMin=[]  NOutMax=[]  SumOutMin=[]  SumOutMax=[]  SaturationOutMin=[]  SaturationOutMax=[]  PParamMin=[]  PParamMax=[]  IParamMin=[]  IParamMax=[]  DParamMin=[]  DParamMax=[]  NParamMin=[]  NParamMax=[]  KbParamMin=[]  KbParamMax=[]  KtParamMin=[]  KtParamMax=[]  KbOutMin=[]  KbOutMax=[]  KtOutMin=[]  KtOutMax=[]  IntegratorOutMin=[]  IntegratorOutMax=[]  FilterOutMin=[]  FilterOutMax=[]  SumI1OutMin=[]  SumI1OutMax=[]  SumI2OutMin=[]  SumI2OutMax=[]  SumI3OutMin=[]  SumI3OutMax=[]  SumI4OutMin=[]  SumI4OutMax=[]  SumDOutMin=[]  SumDOutMax=[]  DifferentiatorOutMin=[]  DifferentiatorOutMax=[]  FilterDiffOutCoefMin=[]  FilterDiffOutCoefMax=[]  ReciprocalOutMin=[]  ReciprocalOutMax=[]  SumDenOutMin=[]  SumDenOutMax=[]  SumNumOutMin=[]  SumNumOutMax=[]  DivideOutMin=[]  DivideOutMax=[]  IntegratorContinuousStateAttributes=''  IntegratorStateMustResolveToSignalObject=off  IntegratorRTWStateStorageClass=Auto  FilterContinuousStateAttributes=''  FilterStateMustResolveToSignalObject=off  FilterRTWStateStorageClass=Auto  ParallelPVariant=InternalParameters  IdealPVariant=Disabled  IVariant=InternalParameters  DVariant=InternalParameters  IntegratorVariant=Discrete  SatVariant=Disabled  AWVariant=Passthrough  PCopyVariant=Disabled  TRVariant=Disabled  FdbkBlocksVariant=Forward  IdealPFdbkVariant=Disabled  SatFdbkVariant=Disabled  DerivativeFilterVariant=ForwardEulerFilter  NVariant=InternalParameters  NCopyVariant=Disabled  FilterICVariant=InternalICsFilter  IntegratorICVariant=InternalICs  ExternalResetVariant=Disabled  TRSumVariant=Passthrough  SumFdbkVariant=Disabled  SumVariant=Sum_PID
  PID Controller3 : simulink/Continuous/PID Controller  Controller=PID  Form=Parallel  TimeDomain=Discrete-time  SampleTime=0.001  IntegratorMethod=Forward Euler  FilterMethod=Forward Euler  ControllerParametersSource=internal  P=40  I=0.1  D=0.5  UseFilter=on  N=200  TunerSelectOption=Transfer Function Based (PID Tuner App)  InitialConditionSource=internal  InitialConditionForIntegrator=0  InitialConditionForFilter=0  DifferentiatorICPrevScaledInput=0  ExternalReset=none  TrackingMode=off  Kt=1  LimitOutput=off  UpperSaturationLimit=inf  LowerSaturationLimit=-inf  LinearizeAsGain=on  AntiWindupMode=none  Kb=1  POutMin=[]  POutMax=[]  IOutMin=[]  IOutMax=[]  DOutMin=[]  DOutMax=[]  NOutMin=[]  NOutMax=[]  SumOutMin=[]  SumOutMax=[]  SaturationOutMin=[]  SaturationOutMax=[]  PParamMin=[]  PParamMax=[]  IParamMin=[]  IParamMax=[]  DParamMin=[]  DParamMax=[]  NParamMin=[]  NParamMax=[]  KbParamMin=[]  KbParamMax=[]  KtParamMin=[]  KtParamMax=[]  KbOutMin=[]  KbOutMax=[]  KtOutMin=[]  KtOutMax=[]  IntegratorOutMin=[]  IntegratorOutMax=[]  FilterOutMin=[]  FilterOutMax=[]  SumI1OutMin=[]  SumI1OutMax=[]  SumI2OutMin=[]  SumI2OutMax=[]  SumI3OutMin=[]  SumI3OutMax=[]  SumI4OutMin=[]  SumI4OutMax=[]  SumDOutMin=[]  SumDOutMax=[]  DifferentiatorOutMin=[]  DifferentiatorOutMax=[]  FilterDiffOutCoefMin=[]  FilterDiffOutCoefMax=[]  ReciprocalOutMin=[]  ReciprocalOutMax=[]  SumDenOutMin=[]  SumDenOutMax=[]  SumNumOutMin=[]  SumNumOutMax=[]  DivideOutMin=[]  DivideOutMax=[]  IntegratorContinuousStateAttributes=''  IntegratorStateMustResolveToSignalObject=off  IntegratorRTWStateStorageClass=Auto  FilterContinuousStateAttributes=''  FilterStateMustResolveToSignalObject=off  FilterRTWStateStorageClass=Auto  ParallelPVariant=InternalParameters  IdealPVariant=Disabled  IVariant=InternalParameters  DVariant=InternalParameters  IntegratorVariant=Discrete  SatVariant=Disabled  AWVariant=Passthrough  PCopyVariant=Disabled  TRVariant=Disabled  FdbkBlocksVariant=Forward  IdealPFdbkVariant=Disabled  SatFdbkVariant=Disabled  DerivativeFilterVariant=ForwardEulerFilter  NVariant=InternalParameters  NCopyVariant=Disabled  FilterICVariant=InternalICsFilter  IntegratorICVariant=InternalICs  ExternalResetVariant=Disabled  TRSumVariant=Passthrough  SumFdbkVariant=Disabled  SumVariant=Sum_PID
  PID Controller5 : simulink/Continuous/PID Controller  Controller=PID  Form=Parallel  TimeDomain=Discrete-time  SampleTime=0.001  IntegratorMethod=Forward Euler  FilterMethod=Forward Euler  ControllerParametersSource=internal  P=20  I=0.1  D=0.5  UseFilter=on  N=200  TunerSelectOption=Transfer Function Based (PID Tuner App)  InitialConditionSource=internal  InitialConditionForIntegrator=0  InitialConditionForFilter=0  DifferentiatorICPrevScaledInput=0  ExternalReset=none  TrackingMode=off  Kt=1  LimitOutput=off  UpperSaturationLimit=inf  LowerSaturationLimit=-inf  LinearizeAsGain=on  AntiWindupMode=none  Kb=1  POutMin=[]  POutMax=[]  IOutMin=[]  IOutMax=[]  DOutMin=[]  DOutMax=[]  NOutMin=[]  NOutMax=[]  SumOutMin=[]  SumOutMax=[]  SaturationOutMin=[]  SaturationOutMax=[]  PParamMin=[]  PParamMax=[]  IParamMin=[]  IParamMax=[]  DParamMin=[]  DParamMax=[]  NParamMin=[]  NParamMax=[]  KbParamMin=[]  KbParamMax=[]  KtParamMin=[]  KtParamMax=[]  KbOutMin=[]  KbOutMax=[]  KtOutMin=[]  KtOutMax=[]  IntegratorOutMin=[]  IntegratorOutMax=[]  FilterOutMin=[]  FilterOutMax=[]  SumI1OutMin=[]  SumI1OutMax=[]  SumI2OutMin=[]  SumI2OutMax=[]  SumI3OutMin=[]  SumI3OutMax=[]  SumI4OutMin=[]  SumI4OutMax=[]  SumDOutMin=[]  SumDOutMax=[]  DifferentiatorOutMin=[]  DifferentiatorOutMax=[]  FilterDiffOutCoefMin=[]  FilterDiffOutCoefMax=[]  ReciprocalOutMin=[]  ReciprocalOutMax=[]  SumDenOutMin=[]  SumDenOutMax=[]  SumNumOutMin=[]  SumNumOutMax=[]  DivideOutMin=[]  DivideOutMax=[]  IntegratorContinuousStateAttributes=''  IntegratorStateMustResolveToSignalObject=off  IntegratorRTWStateStorageClass=Auto  FilterContinuousStateAttributes=''  FilterStateMustResolveToSignalObject=off  FilterRTWStateStorageClass=Auto  ParallelPVariant=InternalParameters  IdealPVariant=Disabled  IVariant=InternalParameters  DVariant=InternalParameters  IntegratorVariant=Discrete  SatVariant=Disabled  AWVariant=Passthrough  PCopyVariant=Disabled  TRVariant=Disabled  FdbkBlocksVariant=Forward  IdealPFdbkVariant=Disabled  SatFdbkVariant=Disabled  DerivativeFilterVariant=ForwardEulerFilter  NVariant=InternalParameters  NCopyVariant=Disabled  FilterICVariant=InternalICsFilter  IntegratorICVariant=InternalICs  ExternalResetVariant=Disabled  TRSumVariant=Passthrough  SumFdbkVariant=Disabled  SumVariant=Sum_PID
  Saturation1 : Saturate  UpperLimit=30  LowerLimit=-30  LinearizeAsGain=off
  Saturation2 : Saturate  UpperLimit=30  LowerLimit=-30  LinearizeAsGain=off
  Saturation3 : Saturate  UpperLimit=30  LowerLimit=-30  LinearizeAsGain=off
  Subsystem : Subsystem
  Rate Demand : Outport
  wires:
  Add2/1 -> PID Controller3/1
  Add3/1 -> PID Controller1/1
  Add1/1 -> PID Controller5/1
  PID Controller5/1 -> Saturation1/1  "Roll_RD"
  PID Controller1/1 -> Saturation3/1  "Yaw_RD"
  PID Controller3/1 -> Saturation2/1  "Pitch_RD"
  Bus Selector1/1 -> Gain2/1  "<Xv>"
  Bus Selector1/2 -> Gain/1  "<Rd>"
  Subsystem/1(Roll) -> Add1/2
  Subsystem/2(Pitch) -> Add2/2
  "States "/1 -> Bus Selector/1
  Bus Selector/1 -> Subsystem/1(Euler)  "<Euler>"
  Subsystem/3(Yaw) -> Add3/2
  "Demand "/1 -> Bus Selector1/1
  Bus Selector1/3 -> Gain1/1  "<Pd>"
  Bus Creator/1 -> Rate Demand/1
  Gain2/1 -> Bus Creator/1  "Z_VD"
  Saturation3/1 -> Bus Creator/4  "Yaw_RD"
  Saturation2/1 -> Bus Creator/3  "Pitch_RD"
  Saturation1/1 -> Bus Creator/2  "Roll_RD"
  Bus Selector1/4 -> Add3/1  "<Yd>"
  Gain/1 -> Add1/1
  Gain1/1 -> Add2/1
